simulink model "AC_Quadcopter_Simulation_BackStepping_ITSE"  (R2015b)
settings: Solver=FixedStepAuto  StartTime=0  StopTime=10  FixedStep=0.02  MaxStep=0.06  RelTol=1e-3
model workspace (MAT data in the model file):
  Sig = Simulink.Signal
  Sig.DataType = 'auto'
  Sig.Units = 'auto'
  Sig.Dimensions = -1
  Sig.DimensionsMode = 'auto'
  Sig.Complexity = 'auto'
  Sig.SampleTime = -1
  Sig.SamplingMode = 'auto'
Description:
  | This is a configurable quadcopter simulation.
  | This Simulink model demonstates attitude control.
  | 
  | Additional quadcopter modeling and simulation materials available at:
  | github.com/dch33/Quad-Sim
  | 
  | Copyright (C) 2014 D. Hartman, K. Landis, S. Moreno, J. Kim, M. Mehrer
  | 
  | License:
  |     This program is free software: you can redistribute it and/or modify
  |     it under the terms of the GNU LESSER GENERAL PUBLIC LICENSE as published by
  |     the Free Software Foundation, either version 3 of the License, or
  |     (at your option) any later version.
  | 
  |     This program is distributed in the hope that it will be useful,
  |     but WITHOUT ANY WARRANTY; without even the implied warranty of
  |     MERCHANTABILITY or FITNESS FOR A PARTICULAR PURPOSE.  See the
  |     GNU General Public License for more details.
  | 
  |     You should have received a copy of the GNU LESSER GENERAL PUBLIC LICENSE
  |     along with this program.  If not, see <http://www.gnu.org/licenses/>.
settings Model: ModifiedComment=HKJ -- Tue Jan 26 08:17:55 2016 -- Version 1.7  Creator=David Hartman  LastModifiedBy=HL
settings Model: ModifiedHistory=|
  | HKJ -- Tue Jan 26 08:17:55 2016 -- Version 1.7
  | 
  | 
  | HKJ -- Tue Jan 26 08:17:55 2016 -- Version 1.7
  | 
  | 
  | HKJ -- Sat Jan 23 14:54:19 2016 -- Version 1.6
  | 
  | 
  | davidhartman -- Fri Jun 06 23:19:51 2014 -- Version 1.5
  | 
  | 
  | davidhartman -- Fri Jun 06 22:53:10 2014 -- Version 1.3
settings SolverCC: AutoInsertRateTranBlk=on
settings DataIOCC: LimitDataPoints=off  SaveFormat=Array  SignalLogging=off  TimeSaveName=btout  OutputSaveName=byout
settings OptimizationCC: DefaultParameterBehavior=Inlined
settings DebuggingCC: UnderspecifiedInitializationDetection=Classic  MergeDetectMultiDrivingBlocksExec=none  SolverPrmCheckMsg=warning  UniqueDataStoreMsg=warning  StateNameClashWarn=warning  StrictBusMsg=WarnOnBusTreatedAsVector
settings HardwareCC: ProdBitPerPointer=32  ProdLargestAtomicFloat=None  ProdIntDivRoundTo=Undefined  ProdEndianess=Unspecified  ProdWordSize=32  ProdHWDeviceType=32-bit Generic
settings GRTTargetCC: GeneratePreprocessorConditionals=Disable all
settings ConfigComp: CovModelRefEnable=Off  CovSFcnEnable=off

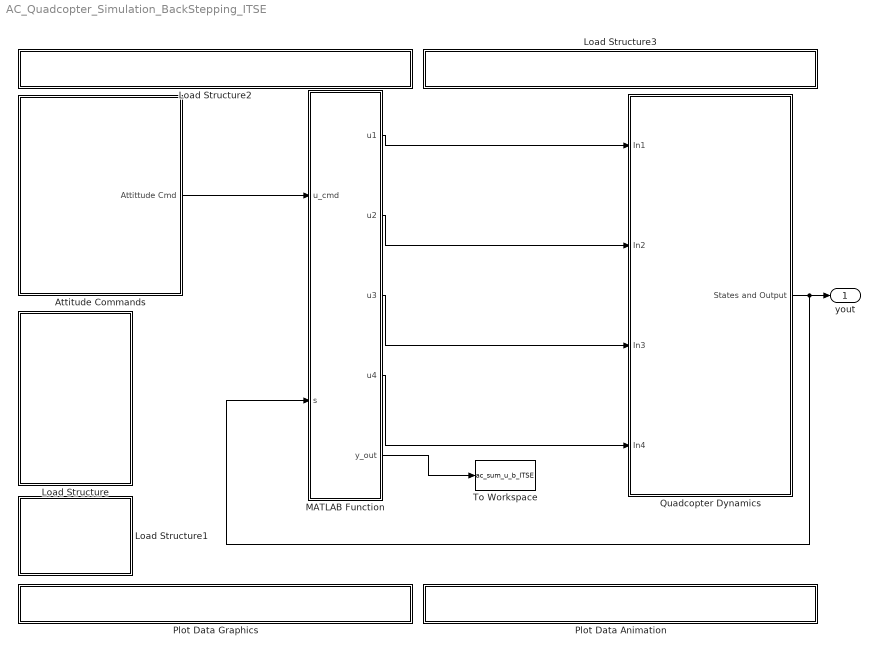
== system AC_Quadcopter_Simulation_BackStepping_ITSE ==
  Attitude Commands : Subsystem
  Load Structure : Subsystem
      settings: OpenFcn=|
      | uiopen('load')
      | if (exist('IC')==1 && exist('quadModel')==1)
      | set_param(bdroot, 'SimulationCommand', 'update')
      | end
      mask Display: fprintf('LOAD:\nQuadcopter\nModel Or\nInitial\nConditions');
  Load Structure1 : Subsystem
      settings: OpenFcn=|
      | if (exist('IC')==1 && exist('quadModel')==1 && exist('yout') && exist('tout'))
      | saveSimResults()
      | else
      | msgbox('No Data To Save!')
      | end
      mask Display: fprintf('SAVE:\nSimulation\nResults');
  Load Structure2 : Subsystem
      settings: OpenFcn=|
      | if exist('GUI_Modeling') == 2,
      | run('GUI_Modeling')
      | 
      | else
      | 
      | msgbox('The desired GUI must be first added to MATLABs path.')
      | 
      | end
      mask Display: fprintf('OPEN GUI: Build New \n Model');
  Load Structure3 : Subsystem
      settings: OpenFcn=|
      | if exist('GUI_IC') == 2,
      | run('GUI_IC')
      | 
      | else
      | 
      | msgbox('The desired GUI must be first added to MATLABs path.')
      | 
      | end
      mask Display: fprintf('OPEN GUI: Create Initial \n Conditions');
  MATLAB Function : MATLAB Function  TreatAsAtomicUnit=on
  Plot Data Animation : Subsystem
      settings: OpenFcn=|
      | if exist('QuadAnim4') == 2,
      |     if exist('yout')
      | 	run('QuadAnim4');
      |     else
      |     msgbox('Simulation must be run before data can be plotted.');
      |     end
      | else                                                                          msgbox('The desired GUI must be first added to MATLABs path.')
      | end
      mask Display: fprintf('OPEN GUI: Flight Animation')
  Plot Data Graphics : Subsystem
      settings: OpenFcn=|
      | if exist('yout')
      | yout = evalin('base', 'yout');
      | tout = evalin('base', 'tout');
      | quadPlots(yout, tout)
      | else
      | msgbox('Simulation must be run before data can be plotted.')
      | end
      mask Display: fprintf('OPEN PLOT: State Data')
  Quadcopter Dynamics : Subsystem
  To Workspace : ToWorkspace  VariableName=ac_sum_u_b_ITSE  SampleTime=-1
  yout : Outport
  wires:
  Quadcopter Dynamics/1(States and Output) -> MATLAB Function/2(s), yout/1
  MATLAB Function/1(u1) -> Quadcopter Dynamics/1(In1)
  MATLAB Function/2(u2) -> Quadcopter Dynamics/2(In2)
  MATLAB Function/3(u3) -> Quadcopter Dynamics/3(In3)
  MATLAB Function/4(u4) -> Quadcopter Dynamics/4(In4)
  Attitude Commands/1(Attittude Cmd) -> MATLAB Function/1(u_cmd)
  MATLAB Function/5(y_out) -> To Workspace/1

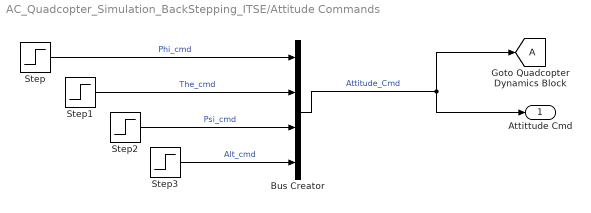
== system AC_Quadcopter_Simulation_BackStepping_ITSE/Attitude Commands ==
  Bus Creator : BusCreator  Inputs=4
  Step : Step  Time=0  After=-15*pi/180  SampleTime=0
  Step1 : Step  Time=0  After=15*pi/180  SampleTime=0
  Step2 : Step  Time=0  After=15*pi/180  SampleTime=0
  Step3 : Step  Time=0  Before=1  SampleTime=0
  Attittude Cmd : Outport
  tag scope: A=global
  wires:
  Bus Creator/1 -> Attittude Cmd/1, [A]  "Attitude_Cmd"
  Step3/1 -> Bus Creator/4  "Alt_cmd"
  Step2/1 -> Bus Creator/3  "Psi_cmd"
  Step1/1 -> Bus Creator/2  "The_cmd"
  Step/1 -> Bus Creator/1  "Phi_cmd"

== system AC_Quadcopter_Simulation_BackStepping_ITSE/Load Structure ==

== system AC_Quadcopter_Simulation_BackStepping_ITSE/Load Structure1 ==

== system AC_Quadcopter_Simulation_BackStepping_ITSE/Load Structure2 ==

== system AC_Quadcopter_Simulation_BackStepping_ITSE/Load Structure3 ==

== system AC_Quadcopter_Simulation_BackStepping_ITSE/Plot Data Animation ==

== system AC_Quadcopter_Simulation_BackStepping_ITSE/Plot Data Graphics ==

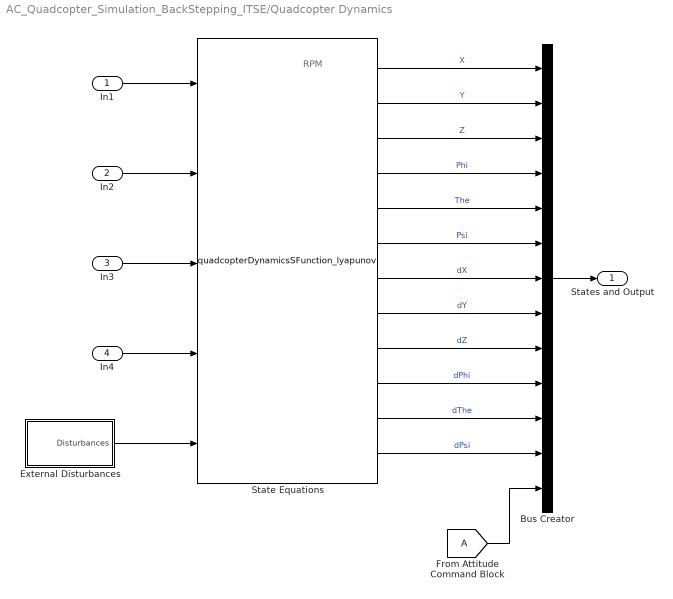
== system AC_Quadcopter_Simulation_BackStepping_ITSE/Quadcopter Dynamics ==
  note: RPM
  In1 : Inport
  In2 : Inport  Port=2
  In3 : Inport  Port=3
  In4 : Inport  Port=4
  Bus Creator : BusCreator  Inputs='X','Y','Z','Phi','The','Psi','dX','dY','dZ','dPhi','dThe','dPsi','Attitude_Cmd'
  External Disturbances : Subsystem
  State Equations : M-S-Function  FunctionName=quadcopterDynamicsSFunction_lyapunov  Parameters=quadModel, IC
      mask Display:
      | port_label('input', 1, 'RPM1')
      | port_label('input', 2, 'RPM2')
      | port_label('input', 3, 'RPM3')
      | port_label('input', 4, 'RPM4')
      | port_label('input', 5, 'Disturbances')
      | port_label('output', 1, 'X')
      | port_label('output', 2, 'Y')
      | port_label('output', 3, 'Z')
      | port_label('output', 4, 'Phi')
      | port_label('output', 5, 'The')
      | port_label('output', 6, 'Psi')
      | port_label('output', 7, 'dX')
      | port_label('output', 8, 'dY')
      | port_label('output', 9, 'dZ')
      | port_label('output', 10, 'dPhi')
      | port_label('output', 11, 'dThe')
      | port_label('output', 12, 'dPsi')
  States and Output : Outport
  wires:
  [A] -> Bus Creator/13
  External Disturbances/1("Disturbances ") -> State Equations/5
  Bus Creator/1 -> States and Output/1
  State Equations/12 -> Bus Creator/12  "dPsi"
  State Equations/11 -> Bus Creator/11  "dThe"
  State Equations/10 -> Bus Creator/10  "dPhi"
  State Equations/9 -> Bus Creator/9  "dZ"
  State Equations/8 -> Bus Creator/8  "dY"
  State Equations/7 -> Bus Creator/7  "dX"
  State Equations/6 -> Bus Creator/6  "Psi"
  State Equations/5 -> Bus Creator/5  "The"
  State Equations/4 -> Bus Creator/4  "Phi"
  State Equations/3 -> Bus Creator/3  "Z"
  State Equations/2 -> Bus Creator/2  "Y"
  State Equations/1 -> Bus Creator/1  "X"
  In4/1 -> State Equations/4
  In3/1 -> State Equations/3
  In2/1 -> State Equations/2
  In1/1 -> State Equations/1

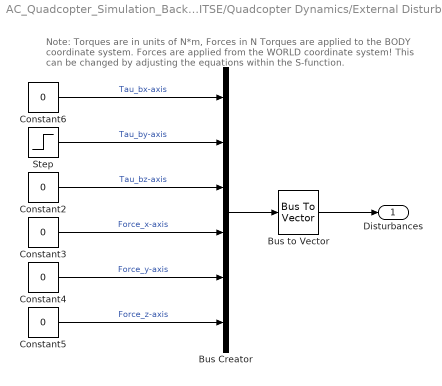
== system AC_Quadcopter_Simulation_BackStepping_ITSE/Quadcopter Dynamics/External Disturbances ==
  note: Note: Torques are in units of N*m, Forces in N
      | Torques are applied to the BODY coordinate system.
      | Forces are applied from the WORLD coordinate system!
      | This can be changed by adjusting the equations within the S-function.
  Bus Creator : BusCreator  Inputs=6
  Bus to Vector : BusToVector
  Constant{2..6} (5 alike) : Constant  Value=0
  Step : Step  After=0  SampleTime=0
  "Disturbances " : Outport
  wires:
  Constant5/1 -> Bus Creator/6  "Force_z-axis"
  Constant4/1 -> Bus Creator/5  "Force_y-axis"
  Constant3/1 -> Bus Creator/4  "Force_x-axis"
  Constant2/1 -> Bus Creator/3  "Tau_bz-axis"
  Step/1 -> Bus Creator/2  "Tau_by-axis"
  Constant6/1 -> Bus Creator/1  "Tau_bx-axis"
  Bus Creator/1 -> Bus to Vector/1
  Bus to Vector/1 -> "Disturbances "/1

== matlab function AC_Quadcopter_Simulation_BackStepping_ITSE/MATLAB Function ==
  data: u_cmd input; u1 output; s input; u2 output; u3 output; u4 output; y_out output
function [u1,u2,u3,u4,y_out] = fcn(u_cmd,s)
k1 = 5;
k2 = 5;
k3 = 5;
k4 = 5;
k5 = 1.5;
k6 = 2;
k7=1;
k8=0.5;

Ix = 0.0094999;Iy=0.0094999;Iz=0.018576;
m=1.023;g=9.81;
L=0.185738;%z这个值有问题

phi_cmd = u_cmd(1);
the_cmd = u_cmd(2);
psi_cmd = u_cmd(3);
alt_cmd = u_cmd(4);

z = s(3);
phi = s(4);the = s(5);psi = s(6);
dz = s(9);
dphi = s(10);dthe = s(11);dpsi = s(12);

e1 = phi-phi_cmd;
e2 = dphi+k1*e1;
e3 = the-the_cmd;
e4 = dthe+k3*e3;
e5 = psi-psi_cmd;
e6 = dpsi+k5*e5;
e7 = z-alt_cmd;
e8 = dz + k7*e7;

u1 = m*(g+(k7^2-1)*e7-(k7+k8)*e8)/(cos(phi)*cos(the));
u2 =Ix/L*(-dthe*dpsi*(Iy-Iz)/Ix+(k1^2-1)*e1-(k1+k2)*e2);
u3 =Iy/L*(-dphi*dpsi*(Iz-Ix)/Iy+(k3^2-1)*e3-(k3+k4)*e4);
u4 =Iz*(-dthe*dphi*(Ix-Iy)/Iz+(k5^2-1)*e5-(k5+k6)*e6);
y_out = u2*u2+u3*u3+u4*u4;
